simulink model "test"  (Simulink 7.6)
settings: Solver=ode45  StartTime=0.0  StopTime=2  RelTol=1e-3
settings Model: Creator=Admin  LastModifiedBy=Admin

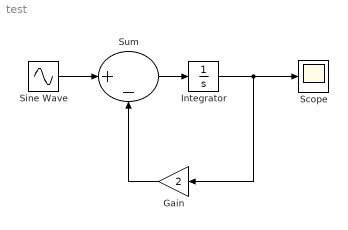
== system test ==
  Gain : Gain  Gain=2
  Integrator : Integrator
  Scope : Scope
  Sine Wave : Sin  SampleTime=0
  Sum : Sum  Inputs=|+-
  wires:
  Sine Wave/1 -> Sum/1
  Sum/1 -> Integrator/1
  Gain/1 -> Sum/2
  Integrator/1 -> Scope/1, Gain/1
